simulink model "impact_angle_control"  (R2024b)
settings: Solver=ode4  StartTime=0.0  StopTime=tf  FixedStep=0.01  RelTol=1e-3
values from neighbouring files (symbols this model uses):
  e0 = lambda0*N - gamma0 - (N - 1)*gamma_T0    [parameters_new.m]
  gamma0 = deg2rad(90)    [parameters_new.m]
  gammaf = -pi/4    (= -0.785398163397)    [parameters_new.m]
  Ki = (0.83/damping_ratio)^2    [parameters_new.m]
  Kp = 2*damping_ratio*sqrt(Ki)    [parameters_new.m]
  main_guidance = 1    [parameters_new.m]
  N = numel(matFiles)    [all_three_scenario_for_impact.m]    (also in parameters_new.m = 1.25)
  r0 = 5000    [parameters_new.m]
  vP = 25    [parameters_new.m]
  xP_initial = 0    [parameters_new.m]
  yP_initial = 0    [parameters_new.m]
settings Model: Creator=AK127381  LastModifiedBy=AK127381

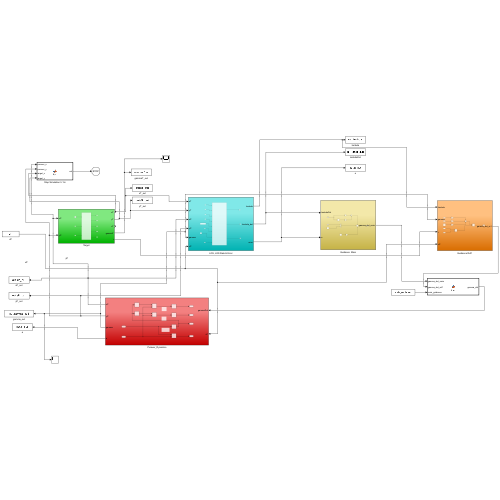
[thumbnail: Simulink's stored preview of the top-level diagram]
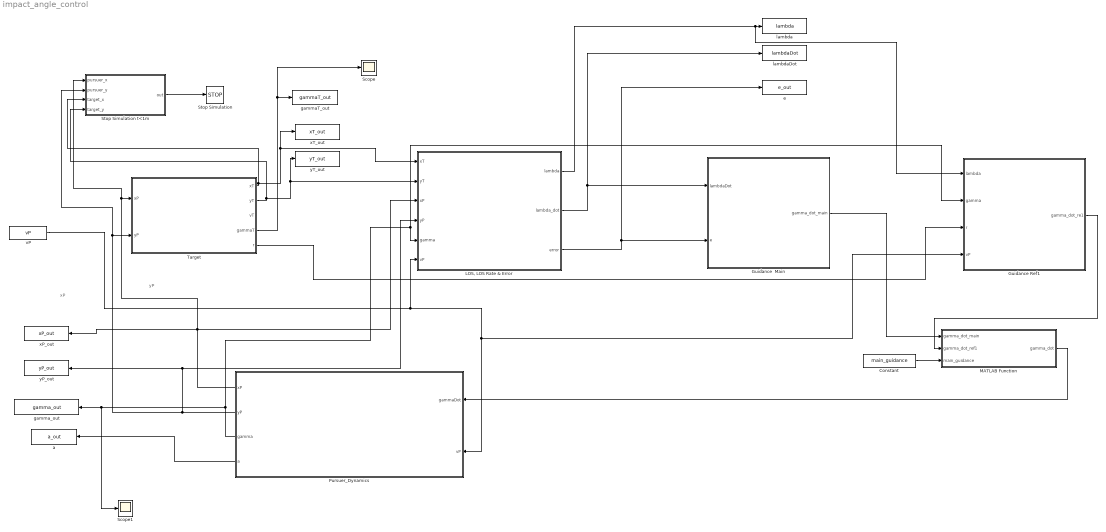
== system impact_angle_control ==
  note: xP
  note: yP
  Constant : Constant  Value=main_guidance
  Guidance  Main : Subsystem
  Guidance Ref1 : Subsystem
  "LOS, LOS Rate & Error" : Subsystem
  MATLAB Function : MATLAB Function  TreatAsAtomicUnit=on
  Pursuer_Dynamics : Subsystem
  Scope : Scope
  Scope1 : Scope
  Stop Simulation : Stop
  Stop Simulation t<1m : MATLAB Function  TreatAsAtomicUnit=on
  Target : Subsystem
  a : ToWorkspace  VariableName=a_out  SampleTime=-1
      settings: Save2DSignal=2-D array (concatenate along first dimension)
  e : ToWorkspace  VariableName=e_out  SampleTime=-1
      settings: Save2DSignal=2-D array (concatenate along first dimension)
  gammaT_out : ToWorkspace  VariableName=gammaT_out  SampleTime=-1
      settings: Save2DSignal=2-D array (concatenate along first dimension)
  gamma_out : ToWorkspace  VariableName=gamma_out  SampleTime=-1
      settings: Save2DSignal=2-D array (concatenate along first dimension)
  lambda : ToWorkspace  VariableName=lambda  SampleTime=-1
      settings: Save2DSignal=2-D array (concatenate along first dimension)
  lambdaDot : ToWorkspace  VariableName=lambdaDot  SampleTime=-1
      settings: Save2DSignal=2-D array (concatenate along first dimension)
  vP : Constant  Value=vP
  xP_out : ToWorkspace  VariableName=xP_out  SampleTime=-1
      settings: Save2DSignal=2-D array (concatenate along first dimension)
  xT_out : ToWorkspace  VariableName=xT_out  SampleTime=-1
      settings: Save2DSignal=2-D array (concatenate along first dimension)
  yP_out : ToWorkspace  VariableName=yP_out  SampleTime=-1
      settings: Save2DSignal=2-D array (concatenate along first dimension)
  yT_out : ToWorkspace  VariableName=yT_out  SampleTime=-1
      settings: Save2DSignal=2-D array (concatenate along first dimension)
  wires:
  Pursuer_Dynamics/1(xP) -> xP_out/1, "LOS, LOS Rate & Error"/3(xP), Stop Simulation t<1m/1(pursuer_x), Target/1(xP)
  "LOS, LOS Rate & Error"/1(lambda) -> Guidance Ref1/1(lambda), lambda/1
  Pursuer_Dynamics/3(gamma) -> Guidance Ref1/2(gamma), "LOS, LOS Rate & Error"/5(gamma), Scope1/1, gamma_out/1
  "LOS, LOS Rate & Error"/3(error) -> Guidance  Main/2(e), e/1
  Pursuer_Dynamics/4(a) -> a/1
  Pursuer_Dynamics/2(yP) -> yP_out/1, "LOS, LOS Rate & Error"/4(yP), Stop Simulation t<1m/2(pursuer_y), Target/2(yP)
  Target/4(gammaT) -> Scope/1, gammaT_out/1
  Target/2(yT) -> Stop Simulation t<1m/4(target_y), yT_out/1, "LOS, LOS Rate & Error"/2(yT)
  vP/1 -> "LOS, LOS Rate & Error"/6(vP), Pursuer_Dynamics/2(vP), Guidance Ref1/4(vP)
  Target/1(xT) -> Stop Simulation t<1m/3(target_x), xT_out/1, "LOS, LOS Rate & Error"/1(xT)
  "LOS, LOS Rate & Error"/2(lambda_dot) -> Guidance  Main/1(lambdaDot), lambdaDot/1
  Guidance Ref1/1(gamma_dot_re1) -> MATLAB Function/2(gamma_dot_ref1)
  Guidance  Main/1(gamma_dot_main) -> MATLAB Function/1(gamma_dot_main)
  MATLAB Function/1(gamma_dot) -> Pursuer_Dynamics/1(gammaDot)
  Stop Simulation t<1m/1(out) -> Stop Simulation/1
  Target/5(r) -> Guidance Ref1/3(r)
  Constant/1 -> MATLAB Function/3(main_guidance)

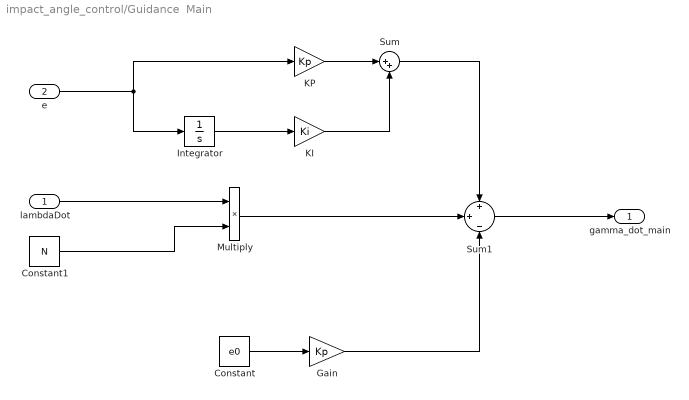
== system impact_angle_control/Guidance  Main ==
  lambdaDot : Inport
  e : Inport  Port=2
  Constant : Constant  Value=e0
  Constant1 : Constant  Value=N
  Gain : Gain  Gain=Kp
  Integrator : Integrator  InitialCondition=e0
  KI : Gain  Gain=Ki
  KP : Gain  Gain=Kp
  Multiply : Product
  Sum : Sum  Inputs=|++
  Sum1 : Sum  Inputs=+|+|-
  gamma_dot_main : Outport
  wires:
  Multiply/1 -> Sum1/2
  Gain/1 -> Sum1/3
  KP/1 -> Sum/1
  Sum1/1 -> gamma_dot_main/1
  Sum/1 -> Sum1/1
  Constant1/1 -> Multiply/2
  Constant/1 -> Gain/1
  Integrator/1 -> KI/1
  e/1 -> KP/1, Integrator/1
  KI/1 -> Sum/2
  lambdaDot/1 -> Multiply/1

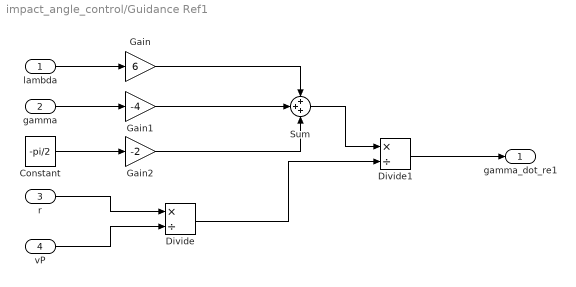
== system impact_angle_control/Guidance Ref1 ==
  lambda : Inport
  gamma : Inport  Port=2
  r : Inport  Port=3
  vP : Inport  Port=4
  Constant : Constant  Value=-pi/2
  Divide : Product  Inputs=*/
  Divide1 : Product  Inputs=*/
  Gain : Gain  Gain=6
  Gain1 : Gain  Gain=-4
  Gain2 : Gain  Gain=-2
  Sum : Sum  Inputs=+++
  gamma_dot_re1 : Outport
  wires:
  lambda/1 -> Gain/1
  gamma/1 -> Gain1/1
  Constant/1 -> Gain2/1
  Gain/1 -> Sum/1
  Gain1/1 -> Sum/2
  Gain2/1 -> Sum/3
  Sum/1 -> Divide1/1
  Divide/1 -> Divide1/2
  r/1 -> Divide/1
  vP/1 -> Divide/2
  Divide1/1 -> gamma_dot_re1/1

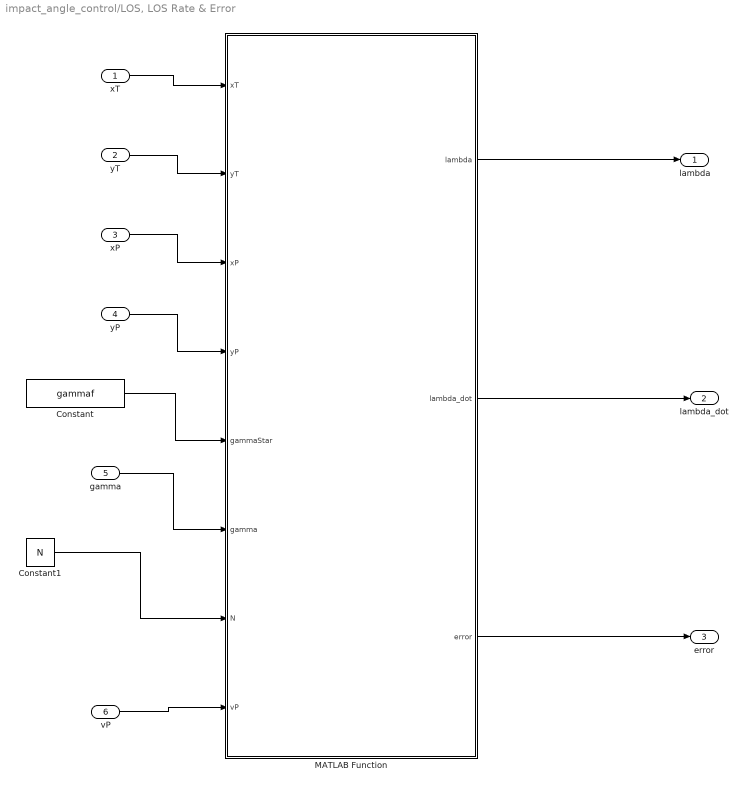
== system impact_angle_control/LOS, LOS Rate & Error ==
  xT : Inport
  yT : Inport  Port=2
  xP : Inport  Port=3
  yP : Inport  Port=4
  gamma : Inport  Port=5
  vP : Inport  Port=6
  Constant : Constant  Value=gammaf
  Constant1 : Constant  Value=N
  MATLAB Function : MATLAB Function  TreatAsAtomicUnit=on
  lambda : Outport
  lambda_dot : Outport  Port=2
  error : Outport  Port=3
  wires:
  xT/1 -> MATLAB Function/1(xT)
  yT/1 -> MATLAB Function/2(yT)
  xP/1 -> MATLAB Function/3(xP)
  yP/1 -> MATLAB Function/4(yP)
  Constant/1 -> MATLAB Function/5(gammaStar)
  MATLAB Function/3(error) -> error/1
  gamma/1 -> MATLAB Function/6(gamma)
  Constant1/1 -> MATLAB Function/7(N)
  MATLAB Function/1(lambda) -> lambda/1
  vP/1 -> MATLAB Function/8(vP)
  MATLAB Function/2(lambda_dot) -> lambda_dot/1

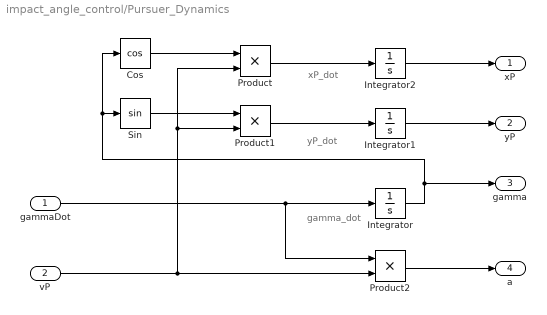
== system impact_angle_control/Pursuer_Dynamics ==
  note: gamma_dot
  note: xP_dot
  note: yP_dot
  gammaDot : Inport
  vP : Inport  Port=2
  Cos : Trigonometry  Operator=cos
  Integrator : Integrator  InitialCondition=gamma0
  Integrator1 : Integrator  InitialCondition=yP_initial
  Integrator2 : Integrator  InitialCondition=xP_initial
  Product : Product
  Product1 : Product
  Product2 : Product
  Sin : Trigonometry
  xP : Outport
  yP : Outport  Port=2
  gamma : Outport  Port=3
  a : Outport  Port=4
  wires:
  vP/1 -> Product/2, Product1/2, Product2/2
  gammaDot/1 -> Integrator/1, Product2/1
  Integrator/1 -> Cos/1, Sin/1, gamma/1
  Integrator2/1 -> xP/1
  Product/1 -> Integrator2/1
  Cos/1 -> Product/1
  Sin/1 -> Product1/1
  Product1/1 -> Integrator1/1
  Integrator1/1 -> yP/1
  Product2/1 -> a/1

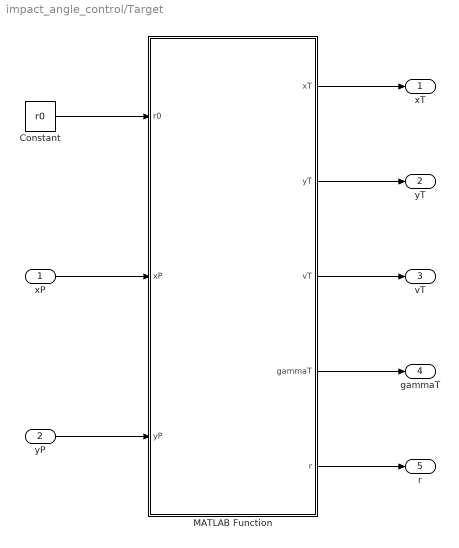
== system impact_angle_control/Target ==
  xP : Inport
  yP : Inport  Port=2
  Constant : Constant  Value=r0
  MATLAB Function : MATLAB Function  TreatAsAtomicUnit=on
  xT : Outport
  yT : Outport  Port=2
  vT : Outport  Port=3
  gammaT : Outport  Port=4
  r : Outport  Port=5
  wires:
  MATLAB Function/1(xT) -> xT/1
  MATLAB Function/2(yT) -> yT/1
  MATLAB Function/3(vT) -> vT/1
  Constant/1 -> MATLAB Function/1(r0)
  MATLAB Function/4(gammaT) -> gammaT/1
  xP/1 -> MATLAB Function/2(xP)
  yP/1 -> MATLAB Function/3(yP)
  MATLAB Function/5(r) -> r/1

== matlab function impact_angle_control/LOS, LOS Rate & Error/MATLAB Function ==
  data: lambda output; xT input; yT input; xP input; yP input; gammaStar input; lambda_dot output; error output; gamma input; N input; vP input
function [ lambda,  lambda_dot, error] = ref1(xT, yT, xP, yP, gammaStar, gamma, N, vP)

    % 1) Relative position
    dx = xT - xP;
    dy = yT - yP;
    
    % 2) Range
    r  = hypot(dx,dy);

    % 3) LOS angle
    lambda = atan2(dy, dx);
    
    % 4) Error term from the paper
    error = N*lambda - gamma - (N-1)*gammaStar;
    
    % 5) Pursuer Velecities
    vPx = cos(gamma)*vP;
    vPy = sin(gamma)*vP;

    % 6) Target Velocities (Which are zero because target is stationary for
    % impact angle control)
    vTx = 0;
    vTy = 0;

    % 7) Relative Velocities
    dvx = vTx - vPx;
    dvy = vTy - vPy;

    % 8) LOS rate
    lambda_dot = (dx*dvy - dy*dvx)/(r*r);
    
end

== matlab function impact_angle_control/Target/MATLAB Function ==
  data: xT output; yT output; vT output; r0 input; gammaT output; r output; xP input; yP input
function [xT, yT, vT, gammaT, r] = targetBlock(r0, xP, yP) 
    
    xT = r0;          
    yT = 0;
    vT = 0;           
    gammaT = -pi/2;
    r = hypot(xT - xP, yT - yP);              

end

== matlab function impact_angle_control/Stop Simulation t<1m ==
  data: pursuer_x input; out output; pursuer_y input; target_x input; target_y input
function out = fcn(pursuer_x, pursuer_y, target_x, target_y)
    % disp('pursuer_x:');
    % disp(pursuer_x);
    % disp('pursuer_y:');
    % disp(pursuer_y);
    % disp('target_x:');
    % disp(target_x);
    % disp('target_y:');
    % disp(target_y);
    % 
    range = sqrt(complex((target_x - pursuer_x)^2 + (target_y - pursuer_y)^2));
    % disp('range:')
    % disp(range)
    % range = target_y - pursuer_y;
    if range < 1
        out = 1;
    else
        out = 0;
    end
end

== matlab function impact_angle_control/MATLAB Function ==
  data: gamma_dot_main input; gamma_dot output; gamma_dot_ref1 input; main_guidance input
function gamma_dot = fcn(gamma_dot_main, gamma_dot_ref1, main_guidance)
    
    if main_guidance== 0
        gamma_dot = gamma_dot_ref1;
        disp('Reference 1 guidance law is engaged')
    else 
        gamma_dot = gamma_dot_main;
        disp( 'main guidance law is engaged')
    end
end
